simulink model "Explicit_MPC"  (R2024b)
settings: Solver=VariableStepAuto  StartTime=0.0  StopTime=30  RelTol=1e-3
libraries: mpclib x1
settings Model: Creator=Reza Shahriari  LastModifiedBy=Reza Shahriari

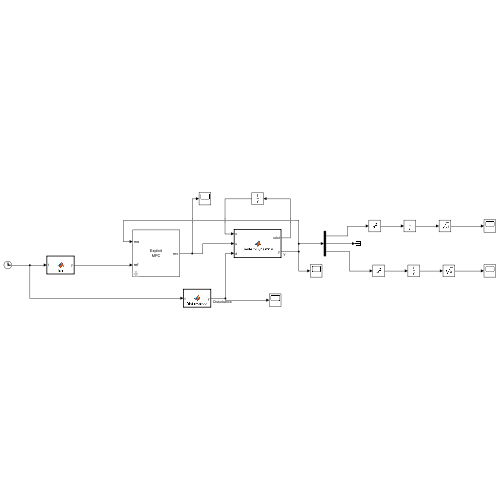
[thumbnail: Simulink's stored preview of the top-level diagram]
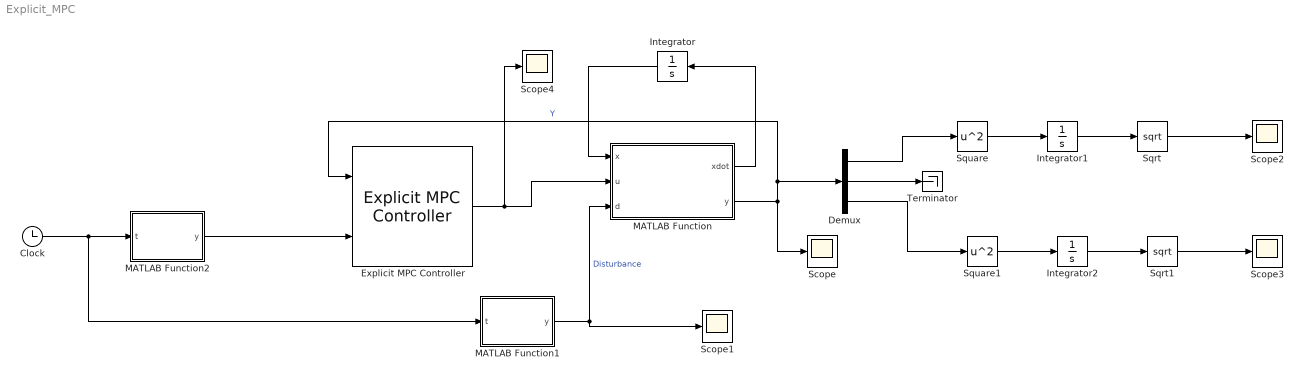
== system Explicit_MPC ==
  Clock : Clock
  Demux : Demux  Outputs=3
  Explicit MPC Controller : mpclib/Explicit MPC Controller  SCDEnableBlockLinearizationSpecification=on  empcobj=explicit  is_multiple=0  enable_value=0  return_u0=off  md_inport=off  mv_inport=off  return_status=off  return_region=off  return_state=off  state_inport=off  BlockDataType=double  SampleTimeInherited=off  switch_inport=off
  Integrator : Integrator  InitialCondition=[0;0;0;0]
  Integrator1 : Integrator
  Integrator2 : Integrator
  MATLAB Function : MATLAB Function  TreatAsAtomicUnit=on
  MATLAB Function1 : MATLAB Function  TreatAsAtomicUnit=on
  MATLAB Function2 : MATLAB Function  TreatAsAtomicUnit=on
  Scope{,1..4} (5 alike) : Scope
  Sqrt : Sqrt
  Sqrt1 : Sqrt
  Square : Math  Operator=square
  Square1 : Math  Operator=square
  Terminator : Terminator
  wires:
  Square/1 -> Integrator1/1
  Square1/1 -> Integrator2/1
  MATLAB Function1/1(y) -> Scope1/1, MATLAB Function/3(d)  "Disturbance"
  Integrator1/1 -> Sqrt/1
  MATLAB Function/2(y) -> Explicit MPC Controller/1, Demux/1, Scope/1  "Y"
  MATLAB Function2/1(y) -> Explicit MPC Controller/2
  Sqrt1/1 -> Scope3/1
  Clock/1 -> MATLAB Function1/1(t), MATLAB Function2/1(t)
  Sqrt/1 -> Scope2/1
  Demux/2 -> Terminator/1
  Demux/1 -> Square/1
  MATLAB Function/1(xdot) -> Integrator/1
  Demux/3 -> Square1/1
  Explicit MPC Controller/1 -> Scope4/1, MATLAB Function/2(u)
  Integrator/1 -> MATLAB Function/1(x)
  Integrator2/1 -> Sqrt1/1

== matlab function Explicit_MPC/MATLAB Function1 ==
  data: t input; y output
function y = Disturbance(t)

if t>=4 & t<5 
    y = t-4;
elseif t>=5 & t<7
    y = 1;
elseif t>=7 & t<8
    y = -t+8;
else 
    y = 0;
end

== matlab function Explicit_MPC/MATLAB Function ==
  data: x input; xdot output; u input; y output; d input
function [xdot,y]= SystemDynamics(x,u,d)

% Parameter Definition
Ms = 2500;
Mu = 320;
ks = 80000;
ku = 500000;
cs = 350;
cu = 15020;

A = [0 1 0 0;
     0 -cs/Ms -ks/Ms cs/Ms;
     0 1 0 -1;
     -ku/Mu cs/Mu (ks+ku)/Mu -(cs+cu)/Mu];
     
B = [0; 1/Ms; 0; -1/Mu];  % Input matrix

C = [1 0 0 0; 0 1 0 0; 0 0 1 0];

Ad = [0.9241    0.0945   -0.0672    0.0013;
   -2.0392    0.8450   -0.6570    0.0178;
    0.8830    0.0843   -0.1675    0.0021;
    1.2927    0.1390   -1.8258   -0.0591];

Bd = [    0.1053;
    2.2534;
   -0.8123;
  -51.0695];

Cd = C;


Diss = [0; cs*cu/(Ms*Mu); -cu/Mu; (cu/Mu)*(ku*cu-cs*Mu-cu*Mu)];

xdot = A*x + B*u + Diss*d;
y = C*x;

== matlab function Explicit_MPC/MATLAB Function2 ==
  data: y output; t input
function y = fcn(t)

y = [0;0;0];
